simulink library "slupdate_aerospace"  (Simulink 4.00)
undefined symbols (not defined in the file or in its folder): g
libraries: aerospace x3, simulink3 x2
settings Model: Creator=sgage  LastModifiedBy=sgage  ExtModeAutoUpdateStatusClock=off

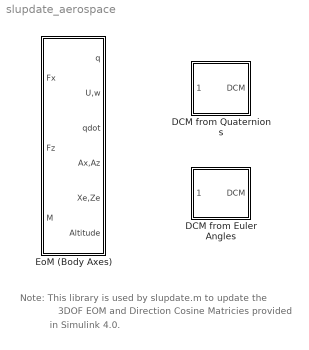
== system slupdate_aerospace ==
  note: 3DOF EOM and Direction Cosine Matricies provided
  note: in Simulink 4.0.
  note: Note: This library is used by slupdate.m to update the
  DCM from Euler Angles : Subsystem
      settings: RTWFcnNameOpts=Auto  RTWFileNameOpts=Auto
      mask Type: Direction Cosine Matrix (R12)
      mask Display: disp('axis')
  DCM from Quaternions : Subsystem
      settings: RTWFcnNameOpts=Auto  RTWFileNameOpts=Auto
      mask Type: Direction Cosine Matrix (R12)
      mask Display: disp('axis')
  EoM (Body Axes) : Subsystem
      settings: RTWFcnNameOpts=Auto  RTWFileNameOpts=Auto
      mask Type: 3 DOF equations of motion (R12)

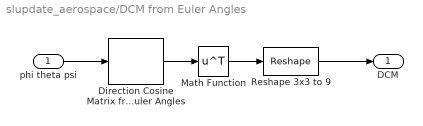
== system slupdate_aerospace/DCM from Euler Angles ==
  phi theta psi : Inport  Port=1  LatchInput=off
  Direction Cosine Matrix from Euler Angles : aerospace/Axes Transformations/Direction Cosine Matrix from Euler Angles
  Math Function : Math  Operator=transpose  OutputSignalType=auto
  Reshape 3x3 to 9 : simulink3/Signals & Systems/Reshape  OutputDimensionality=Customize  OutputDimensions=9
  DCM : Outport  Port=1
  wires:
  phi theta psi/1 -> Direction Cosine Matrix from Euler Angles/1
  Direction Cosine Matrix from Euler Angles/1 -> Math Function/1
  Math Function/1 -> Reshape 3x3 to 9/1
  Reshape 3x3 to 9/1 -> DCM/1

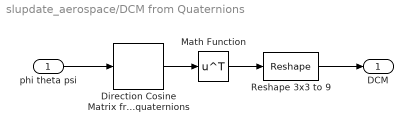
== system slupdate_aerospace/DCM from Quaternions ==
  phi theta psi : Inport  Port=1  LatchInput=off
  Direction Cosine Matrix from quaternions : aerospace/Axes Transformations/Direction Cosine Matrix from quaternions
  Math Function : Math  Operator=transpose  OutputSignalType=auto
  Reshape 3x3 to 9 : simulink3/Signals & Systems/Reshape  OutputDimensionality=Customize  OutputDimensions=9
  DCM : Outport  Port=1
  wires:
  phi theta psi/1 -> Direction Cosine Matrix from quaternions/1
  Direction Cosine Matrix from quaternions/1 -> Math Function/1
  Math Function/1 -> Reshape 3x3 to 9/1
  Reshape 3x3 to 9/1 -> DCM/1

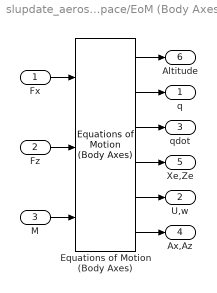
== system slupdate_aerospace/EoM (Body Axes) ==
  Fx : Inport  Port=1  LatchInput=off
  Fz : Inport  Port=2  LatchInput=off
  M : Inport  Port=3  LatchInput=off
  " Equations of Motion (Body Axes)" : aerospace/3DoF Equations of Motion / Equations of Motion (Body Axes)  v_ini=v_ini  theta_ini=theta_ini  alpha_ini=alpha_ini  q_ini=q_ini  pos_ini=pos_ini  mass=mass  Iyy=Iyy  g=g
  q : Outport  Port=1
  U,w : Outport  Port=2
  qdot : Outport  Port=3
  Ax,Az : Outport  Port=4
  Xe,Ze : Outport  Port=5
  Altitude : Outport  Port=6
  wires:
  " Equations of Motion (Body Axes)"/1 -> Altitude/1
  " Equations of Motion (Body Axes)"/4 -> Xe,Ze/1
  " Equations of Motion (Body Axes)"/5 -> U,w/1
  " Equations of Motion (Body Axes)"/6 -> Ax,Az/1
  " Equations of Motion (Body Axes)"/2 -> q/1
  M/1 -> " Equations of Motion (Body Axes)"/3
  Fz/1 -> " Equations of Motion (Body Axes)"/2
  " Equations of Motion (Body Axes)"/3 -> qdot/1
  Fx/1 -> " Equations of Motion (Body Axes)"/1
